simulink model "single_camera_xy_tracking"  (R2025b)
settings: Solver=FixedStepDiscrete  StartTime=0  StopTime=T_end  FixedStep=Ts  RelTol=1e-3
InitFcn:
  | init_single_camera_xy_tracking;
values from neighbouring files (symbols this model uses):
  controller_parameters = [      Ts; Z_hat; Kpx; Kpy; k_ff; gamma_adapt; sigma_adapt; adapt_max;      v_xy_max; a_xy_max; ekf_gate_threshold;      double(enable_proportional); double(enable_ekf_feedforward);      double(enable_adaptation); double(controller_enable);      ekf_reset_timeout_sec]    [init_single_camera_xy_tracking.m]
  cx = 1920    [init_single_camera_xy_tracking.m]
  cy = 1080    [init_single_camera_xy_tracking.m]
  fx = 800    [init_single_camera_xy_tracking.m]
  fy = 800    [init_single_camera_xy_tracking.m]
  joint_state_timeout_sec = 0.10    (= 0.1)    [init_single_camera_xy_tracking.m]
  P0 = diag([0.05^2, 0.05^2, 0.20^2, 0.20^2, 0.50^2, 0.50^2])    [init_single_camera_xy_tracking.m]
  pixel_noise_std = 0.8    [init_single_camera_xy_tracking.m]
  Q_ekf = diag([1e-6, 1e-6, 1e-4, 1e-4, 1e-2, 1e-2])    [init_single_camera_xy_tracking.m]
  R_ekf = diag([0.003^2, 0.003^2])    [init_single_camera_xy_tracking.m]
  random_seed_x = 1207    [init_single_camera_xy_tracking.m]
  random_seed_y = 9053    [init_single_camera_xy_tracking.m]
  target_timeout_sec = 0.20    (= 0.2)    [init_single_camera_xy_tracking.m]
  Ts = 0.01    [init_single_camera_xy_tracking.m]
  USE_ROS = true    [init_single_camera_xy_tracking.m]
  X0 = 0.45    [init_single_camera_xy_tracking.m]
  Y0 = -0.25    [init_single_camera_xy_tracking.m]
  Z0 = Z_hat    (= 0.75)    [init_single_camera_xy_tracking.m]
  Z_hat = 0.75    [init_single_camera_xy_tracking.m]
undefined symbols (not defined in the file or in its folder): data, data_SL_Info
libraries: ros2lib x4
Description:
  | Fixed-focus monocular XY target tracking. Outputs camera-frame [vx vy 0 0 0 0]; robot kinematics remain external.
settings Model: Creator=ASUS  LastModifiedBy=ASUS
settings DataIOCC: SignalLogging=off

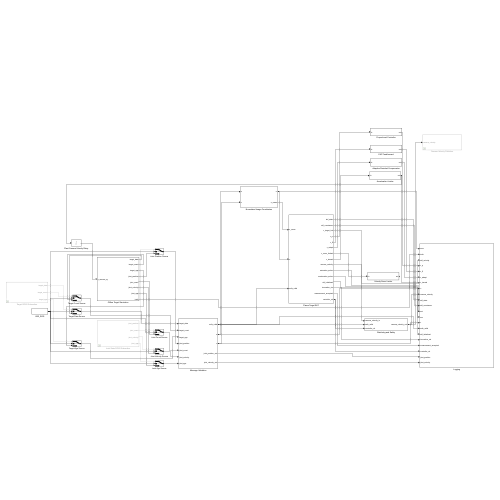
[thumbnail: Simulink's stored preview of the top-level diagram]
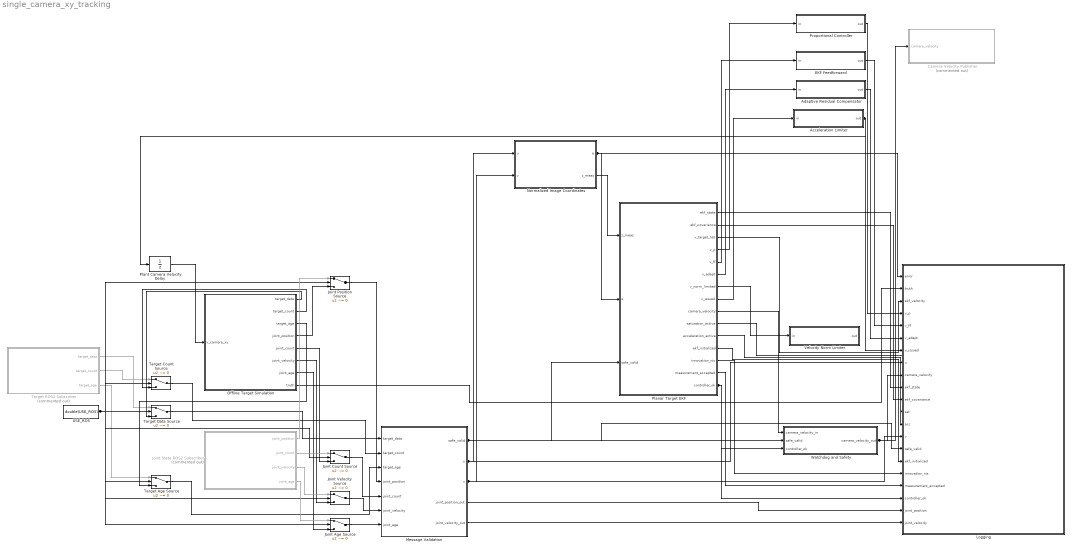
== system single_camera_xy_tracking ==
  Acceleration Limiter : Subsystem
  Adaptive Residual Compensator : Subsystem
  Camera Velocity Publisher : Subsystem  Commented=on
  EKF Feedforward : Subsystem
  Joint Age Source : Switch  Criteria=u2 ~= 0  Threshold=0.5  SaturateOnIntegerOverflow=off  InputSameDT=off
  Joint Count Source : Switch  Criteria=u2 ~= 0  Threshold=0.5  SaturateOnIntegerOverflow=off  InputSameDT=off
  Joint Position Source : Switch  Criteria=u2 ~= 0  Threshold=0.5  SaturateOnIntegerOverflow=off  InputSameDT=off
  Joint State ROS2 Subscriber : Subsystem  Commented=on
  Joint Velocity Source : Switch  Criteria=u2 ~= 0  Threshold=0.5  SaturateOnIntegerOverflow=off  InputSameDT=off
  Logging : Subsystem
  Message Validation : Subsystem
  Normalized Image Coordinates : Subsystem
  Offline Target Simulation : Subsystem
  Planar Target EKF : Subsystem
  Plant Camera Velocity Delay : UnitDelay  InitialCondition=[0;0]  SampleTime=Ts  HasFrameUpgradeWarning=on
  Proportional Controller : Subsystem
  Target Age Source : Switch  Criteria=u2 ~= 0  Threshold=0.5  SaturateOnIntegerOverflow=off  InputSameDT=off
  Target Count Source : Switch  Criteria=u2 ~= 0  Threshold=0.5  SaturateOnIntegerOverflow=off  InputSameDT=off
  Target Data Source : Switch  Criteria=u2 ~= 0  Threshold=0.5  SaturateOnIntegerOverflow=off  InputSameDT=off
  Target ROS2 Subscriber : Subsystem  Commented=on
  USE_ROS : Constant  Value=double(USE_ROS)
  Velocity Norm Limiter : Subsystem
  Watchdog and Safety : Subsystem
  wires:
  Target Age Source/1 -> Message Validation/3(target_age)
  Target Data Source/1 -> Message Validation/1(target_data)
  Target Count Source/1 -> Message Validation/2(target_count)
  Plant Camera Velocity Delay/1 -> Offline Target Simulation/1(v_camera_xy)
  Target ROS2 Subscriber/1(target_data) -> Target Data Source/1
  Planar Target EKF/3(v_target_hat) -> Logging/3(ekf_velocity)
  Message Validation/2(u) -> Logging/8(u), Normalized Image Coordinates/1(u)
  Target ROS2 Subscriber/2(target_count) -> Target Count Source/1
  Target ROS2 Subscriber/3(target_age) -> Target Age Source/1
  Planar Target EKF/15(controller_ok) -> Watchdog and Safety/3(controller_ok), Logging/19(controller_ok)
  Planar Target EKF/7(v_norm_limited) -> Velocity Norm Limiter/1(in)
  USE_ROS/1 -> Joint Age Source/2, Joint Velocity Source/2, Joint Position Source/2, Target Count Source/2, Joint Count Source/2, Target Data Source/2, Target Age Source/2
  Offline Target Simulation/1(target_data) -> Target Data Source/3
  Offline Target Simulation/2(target_count) -> Target Count Source/3
  Offline Target Simulation/3(target_age) -> Target Age Source/3
  Offline Target Simulation/4(joint_position) -> Joint Position Source/3
  Offline Target Simulation/5(joint_count) -> Joint Count Source/3
  Offline Target Simulation/6(joint_velocity) -> Joint Velocity Source/3
  Adaptive Residual Compensator/1(out) -> Logging/6(v_adapt)
  Offline Target Simulation/7(joint_age) -> Joint Age Source/3
  Offline Target Simulation/8(truth) -> Logging/2(truth)
  Joint Age Source/1 -> Message Validation/7(joint_age)
  Joint State ROS2 Subscriber/1(joint_position) -> Joint Position Source/1
  Joint Count Source/1 -> Message Validation/5(joint_count)
  Joint State ROS2 Subscriber/2(joint_count) -> Joint Count Source/1
  Joint Position Source/1 -> Message Validation/4(joint_position)
  Joint State ROS2 Subscriber/3(joint_velocity) -> Joint Velocity Source/1
  Joint State ROS2 Subscriber/4(joint_age) -> Joint Age Source/1
  Joint Velocity Source/1 -> Message Validation/6(joint_velocity)
  Planar Target EKF/4(v_p) -> Proportional Controller/1(in)
  Message Validation/1(safe_valid) -> Watchdog and Safety/2(safe_valid), Logging/15(safe_valid), Planar Target EKF/3(safe_valid)
  Message Validation/3(v) -> Logging/14(v), Normalized Image Coordinates/2(v)
  Planar Target EKF/5(v_ff) -> EKF Feedforward/1(in)
  Message Validation/4(joint_position_out) -> Logging/20(joint_position)
  Message Validation/5(joint_velocity_out) -> Logging/21(joint_velocity)
  Normalized Image Coordinates/1(e) -> Planar Target EKF/2(e), Logging/1(error)
  Normalized Image Coordinates/2(z_meas) -> Planar Target EKF/1(z_meas)
  Planar Target EKF/1(ekf_state) -> Logging/10(ekf_state)
  Planar Target EKF/2(ekf_covariance) -> Logging/11(ekf_covariance)
  Planar Target EKF/14(measurement_accepted) -> Logging/18(measurement_accepted)
  Planar Target EKF/6(v_adapt) -> Adaptive Residual Compensator/1(in)
  Planar Target EKF/8(v_issued) -> Acceleration Limiter/1(in)
  Planar Target EKF/10(saturation_active) -> Logging/12(sat)
  Planar Target EKF/11(acceleration_active) -> Logging/13(acc)
  Planar Target EKF/12(ekf_initialized) -> Logging/16(ekf_initialized)
  Planar Target EKF/13(innovation_nis) -> Logging/17(innovation_nis)
  Proportional Controller/1(out) -> Logging/4(v_p)
  EKF Feedforward/1(out) -> Logging/5(v_ff)
  Acceleration Limiter/1(out) -> Logging/7(v_issued), Plant Camera Velocity Delay/1
  Planar Target EKF/9(camera_velocity) -> Watchdog and Safety/1(camera_velocity_in)
  Watchdog and Safety/1(camera_velocity_out) -> Camera Velocity Publisher/1(camera_velocity), Logging/9(camera_velocity)

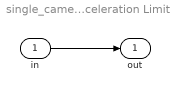
== system single_camera_xy_tracking/Acceleration Limiter ==
  in : Inport
  out : Outport
  wires:
  in/1 -> out/1

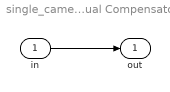
== system single_camera_xy_tracking/Adaptive Residual Compensator ==
  in : Inport
  out : Outport
  wires:
  in/1 -> out/1

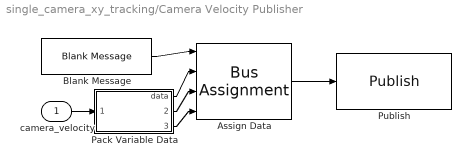
== system single_camera_xy_tracking/Camera Velocity Publisher ==
  camera_velocity : Inport
  Assign Data : BusAssignment  AssignedSignals=data,data_SL_Info.CurrentLength,data_SL_Info.ReceivedLength
  Blank Message : ros2lib/Blank Message  messageClass=Message  entityType=std_msgs/Float64MultiArray  messageType=std_msgs/Float64MultiArray  SampleTime=Ts
  Pack Variable Data : MATLAB Function  TreatAsAtomicUnit=on
  Publish : ros2lib/Publish  topicSource=Select from ROS network  topic=/simulink/camera_velocity  messageType=std_msgs/Float64MultiArray  QOSHistory=Keep last  QOSDepth=1  QOSReliability=Reliable  QOSDurability=Volatile  QOSDeadline=Inf  QOSLifespan=Inf  QOSLiveliness=Automatic  QOSLeaseDuration=Inf  QOSAvoidROSNamespaceConventions=off
  wires:
  Blank Message/1 -> Assign Data/1
  Assign Data/1 -> Publish/1
  camera_velocity/1 -> Pack Variable Data/1(camera_velocity)
  Pack Variable Data/1(data) -> Assign Data/2
  Pack Variable Data/2(current_length) -> Assign Data/3
  Pack Variable Data/3(received_length) -> Assign Data/4

== system single_camera_xy_tracking/EKF Feedforward ==
  in : Inport
  out : Outport
  wires:
  in/1 -> out/1

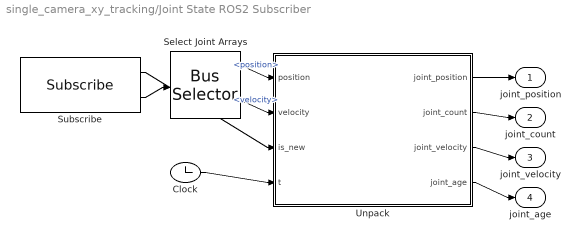
== system single_camera_xy_tracking/Joint State ROS2 Subscriber ==
  Clock : Clock
  Select Joint Arrays : BusSelector  OutputSignals=position,velocity
  Subscribe : ros2lib/Subscribe  topicSource=Select from ROS network  topic=/franka/joint_states  messageType=sensor_msgs/JointState  sampleTime=Ts  QOSHistory=Keep last  QOSDepth=1  QOSReliability=Best effort  QOSDurability=Volatile  QOSDeadline=Inf  QOSLifespan=Inf  QOSLiveliness=Automatic  QOSLeaseDuration=Inf  QOSAvoidROSNamespaceConventions=off
  Unpack : MATLAB Function  TreatAsAtomicUnit=on
  joint_position : Outport
  joint_count : Outport  Port=2
  joint_velocity : Outport  Port=3
  joint_age : Outport  Port=4
  wires:
  Unpack/1(joint_position) -> joint_position/1
  Unpack/2(joint_count) -> joint_count/1
  Unpack/3(joint_velocity) -> joint_velocity/1
  Unpack/4(joint_age) -> joint_age/1
  Select Joint Arrays/1 -> Unpack/1(position)  "<position>"
  Select Joint Arrays/2 -> Unpack/2(velocity)  "<velocity>"
  Clock/1 -> Unpack/4(t)
  Subscribe/2 -> Select Joint Arrays/1
  Subscribe/1 -> Unpack/3(is_new)

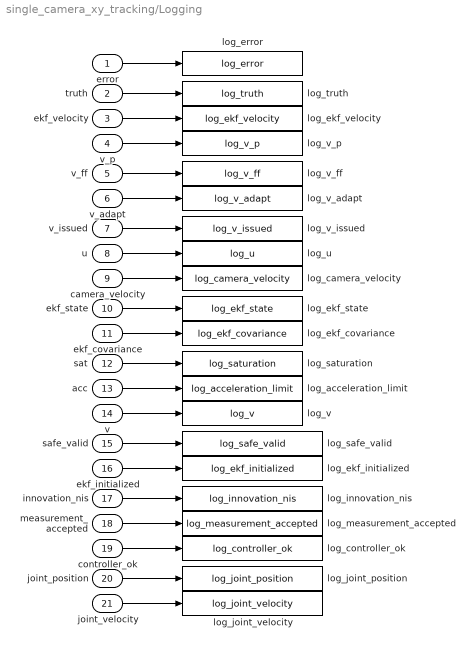
== system single_camera_xy_tracking/Logging ==
  error : Inport
  truth : Inport  Port=2
  ekf_velocity : Inport  Port=3
  v_p : Inport  Port=4
  v_ff : Inport  Port=5
  v_adapt : Inport  Port=6
  v_issued : Inport  Port=7
  u : Inport  Port=8
  camera_velocity : Inport  Port=9
  ekf_state : Inport  Port=10
  ekf_covariance : Inport  Port=11
  sat : Inport  Port=12
  acc : Inport  Port=13
  v : Inport  Port=14
  safe_valid : Inport  Port=15
  ekf_initialized : Inport  Port=16
  innovation_nis : Inport  Port=17
  measurement_accepted : Inport  Port=18
  controller_ok : Inport  Port=19
  joint_position : Inport  Port=20
  joint_velocity : Inport  Port=21
  log_acceleration_limit : ToWorkspace  VariableName=log_acceleration_limit  SaveFormat=Structure With Time  SampleTime=-1
  log_camera_velocity : ToWorkspace  VariableName=log_camera_velocity  SaveFormat=Structure With Time  SampleTime=-1
  log_controller_ok : ToWorkspace  VariableName=log_controller_ok  SaveFormat=Structure With Time  SampleTime=-1
  log_ekf_covariance : ToWorkspace  VariableName=log_ekf_covariance  SaveFormat=Structure With Time  SampleTime=-1
  log_ekf_initialized : ToWorkspace  VariableName=log_ekf_initialized  SaveFormat=Structure With Time  SampleTime=-1
  log_ekf_state : ToWorkspace  VariableName=log_ekf_state  SaveFormat=Structure With Time  SampleTime=-1
  log_ekf_velocity : ToWorkspace  VariableName=log_ekf_velocity  SaveFormat=Structure With Time  SampleTime=-1
  log_error : ToWorkspace  VariableName=log_error  SaveFormat=Structure With Time  SampleTime=-1
  log_innovation_nis : ToWorkspace  VariableName=log_innovation_nis  SaveFormat=Structure With Time  SampleTime=-1
  log_joint_position : ToWorkspace  VariableName=log_joint_position  SaveFormat=Structure With Time  SampleTime=-1
  log_joint_velocity : ToWorkspace  VariableName=log_joint_velocity  SaveFormat=Structure With Time  SampleTime=-1
  log_measurement_accepted : ToWorkspace  VariableName=log_measurement_accepted  SaveFormat=Structure With Time  SampleTime=-1
  log_safe_valid : ToWorkspace  VariableName=log_safe_valid  SaveFormat=Structure With Time  SampleTime=-1
  log_saturation : ToWorkspace  VariableName=log_saturation  SaveFormat=Structure With Time  SampleTime=-1
  log_truth : ToWorkspace  VariableName=log_truth  SaveFormat=Structure With Time  SampleTime=-1
  log_u : ToWorkspace  VariableName=log_u  SaveFormat=Structure With Time  SampleTime=-1
  log_v : ToWorkspace  VariableName=log_v  SaveFormat=Structure With Time  SampleTime=-1
  log_v_adapt : ToWorkspace  VariableName=log_v_adapt  SaveFormat=Structure With Time  SampleTime=-1
  log_v_ff : ToWorkspace  VariableName=log_v_ff  SaveFormat=Structure With Time  SampleTime=-1
  log_v_issued : ToWorkspace  VariableName=log_v_issued  SaveFormat=Structure With Time  SampleTime=-1
  log_v_p : ToWorkspace  VariableName=log_v_p  SaveFormat=Structure With Time  SampleTime=-1
  wires:
  error/1 -> log_error/1
  truth/1 -> log_truth/1
  ekf_velocity/1 -> log_ekf_velocity/1
  v_p/1 -> log_v_p/1
  v_ff/1 -> log_v_ff/1
  v_adapt/1 -> log_v_adapt/1
  v_issued/1 -> log_v_issued/1
  u/1 -> log_u/1
  camera_velocity/1 -> log_camera_velocity/1
  ekf_state/1 -> log_ekf_state/1
  ekf_covariance/1 -> log_ekf_covariance/1
  sat/1 -> log_saturation/1
  acc/1 -> log_acceleration_limit/1
  v/1 -> log_v/1
  safe_valid/1 -> log_safe_valid/1
  ekf_initialized/1 -> log_ekf_initialized/1
  innovation_nis/1 -> log_innovation_nis/1
  measurement_accepted/1 -> log_measurement_accepted/1
  controller_ok/1 -> log_controller_ok/1
  joint_position/1 -> log_joint_position/1
  joint_velocity/1 -> log_joint_velocity/1

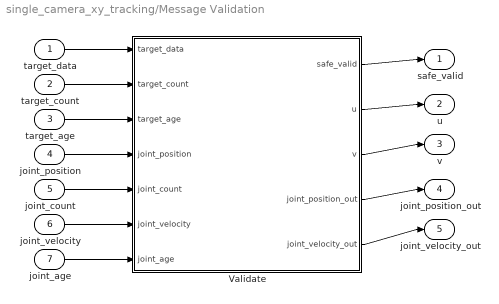
== system single_camera_xy_tracking/Message Validation ==
  target_data : Inport
  target_count : Inport  Port=2
  target_age : Inport  Port=3
  joint_position : Inport  Port=4
  joint_count : Inport  Port=5
  joint_velocity : Inport  Port=6
  joint_age : Inport  Port=7
  Validate : MATLAB Function  TreatAsAtomicUnit=on
  safe_valid : Outport
  u : Outport  Port=2
  v : Outport  Port=3
  joint_position_out : Outport  Port=4
  joint_velocity_out : Outport  Port=5
  wires:
  Validate/1(safe_valid) -> safe_valid/1
  Validate/2(u) -> u/1
  Validate/3(v) -> v/1
  Validate/4(joint_position_out) -> joint_position_out/1
  Validate/5(joint_velocity_out) -> joint_velocity_out/1
  target_data/1 -> Validate/1(target_data)
  target_count/1 -> Validate/2(target_count)
  target_age/1 -> Validate/3(target_age)
  joint_position/1 -> Validate/4(joint_position)
  joint_count/1 -> Validate/5(joint_count)
  joint_velocity/1 -> Validate/6(joint_velocity)
  joint_age/1 -> Validate/7(joint_age)

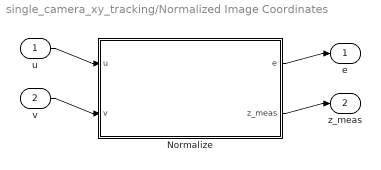
== system single_camera_xy_tracking/Normalized Image Coordinates ==
  u : Inport
  v : Inport  Port=2
  Normalize : MATLAB Function  TreatAsAtomicUnit=on
  e : Outport
  z_meas : Outport  Port=2
  wires:
  u/1 -> Normalize/1(u)
  v/1 -> Normalize/2(v)
  Normalize/1(e) -> e/1
  Normalize/2(z_meas) -> z_meas/1

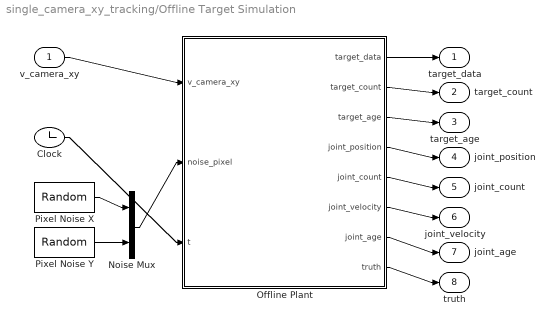
== system single_camera_xy_tracking/Offline Target Simulation ==
  v_camera_xy : Inport
  Clock : Clock
  Noise Mux : Mux  Inputs=2
  Offline Plant : MATLAB Function  TreatAsAtomicUnit=on
  Pixel Noise X : RandomNumber  Variance=pixel_noise_std^2  Seed=random_seed_x  SampleTime=Ts
  Pixel Noise Y : RandomNumber  Variance=pixel_noise_std^2  Seed=random_seed_y  SampleTime=Ts
  target_data : Outport
  target_count : Outport  Port=2
  target_age : Outport  Port=3
  joint_position : Outport  Port=4
  joint_count : Outport  Port=5
  joint_velocity : Outport  Port=6
  joint_age : Outport  Port=7
  truth : Outport  Port=8
  wires:
  Offline Plant/1(target_data) -> target_data/1
  Offline Plant/2(target_count) -> target_count/1
  Offline Plant/3(target_age) -> target_age/1
  Offline Plant/4(joint_position) -> joint_position/1
  Offline Plant/5(joint_count) -> joint_count/1
  Offline Plant/6(joint_velocity) -> joint_velocity/1
  Offline Plant/7(joint_age) -> joint_age/1
  Offline Plant/8(truth) -> truth/1
  v_camera_xy/1 -> Offline Plant/1(v_camera_xy)
  Pixel Noise X/1 -> Noise Mux/1
  Pixel Noise Y/1 -> Noise Mux/2
  Noise Mux/1 -> Offline Plant/2(noise_pixel)
  Clock/1 -> Offline Plant/3(t)

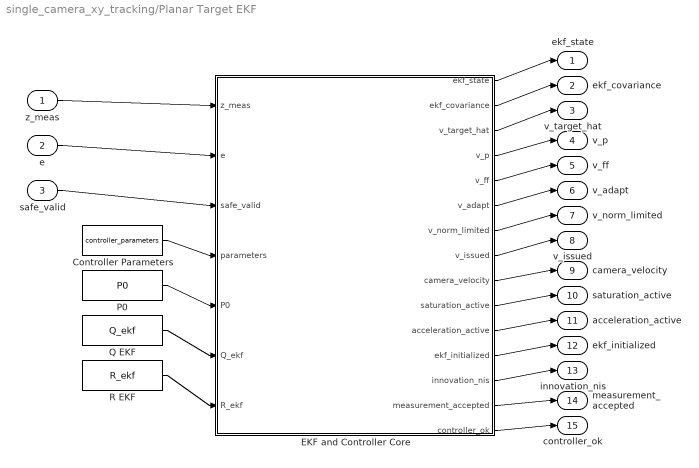
== system single_camera_xy_tracking/Planar Target EKF ==
  z_meas : Inport
  e : Inport  Port=2
  safe_valid : Inport  Port=3
  Controller Parameters : Constant  Value=controller_parameters
  EKF and Controller Core : MATLAB Function  TreatAsAtomicUnit=on
  P0 : Constant  Value=P0
  Q EKF : Constant  Value=Q_ekf
  R EKF : Constant  Value=R_ekf
  ekf_state : Outport
  ekf_covariance : Outport  Port=2
  v_target_hat : Outport  Port=3
  v_p : Outport  Port=4
  v_ff : Outport  Port=5
  v_adapt : Outport  Port=6
  v_norm_limited : Outport  Port=7
  v_issued : Outport  Port=8
  camera_velocity : Outport  Port=9
  saturation_active : Outport  Port=10
  acceleration_active : Outport  Port=11
  ekf_initialized : Outport  Port=12
  innovation_nis : Outport  Port=13
  measurement_accepted : Outport  Port=14
  controller_ok : Outport  Port=15
  wires:
  EKF and Controller Core/1(ekf_state) -> ekf_state/1
  EKF and Controller Core/2(ekf_covariance) -> ekf_covariance/1
  EKF and Controller Core/3(v_target_hat) -> v_target_hat/1
  EKF and Controller Core/4(v_p) -> v_p/1
  EKF and Controller Core/5(v_ff) -> v_ff/1
  EKF and Controller Core/6(v_adapt) -> v_adapt/1
  EKF and Controller Core/7(v_norm_limited) -> v_norm_limited/1
  EKF and Controller Core/8(v_issued) -> v_issued/1
  EKF and Controller Core/9(camera_velocity) -> camera_velocity/1
  EKF and Controller Core/10(saturation_active) -> saturation_active/1
  EKF and Controller Core/11(acceleration_active) -> acceleration_active/1
  EKF and Controller Core/12(ekf_initialized) -> ekf_initialized/1
  EKF and Controller Core/13(innovation_nis) -> innovation_nis/1
  EKF and Controller Core/14(measurement_accepted) -> measurement_accepted/1
  EKF and Controller Core/15(controller_ok) -> controller_ok/1
  z_meas/1 -> EKF and Controller Core/1(z_meas)
  e/1 -> EKF and Controller Core/2(e)
  safe_valid/1 -> EKF and Controller Core/3(safe_valid)
  Controller Parameters/1 -> EKF and Controller Core/4(parameters)
  P0/1 -> EKF and Controller Core/5(P0)
  Q EKF/1 -> EKF and Controller Core/6(Q_ekf)
  R EKF/1 -> EKF and Controller Core/7(R_ekf)

== system single_camera_xy_tracking/Proportional Controller ==
  in : Inport
  out : Outport
  wires:
  in/1 -> out/1

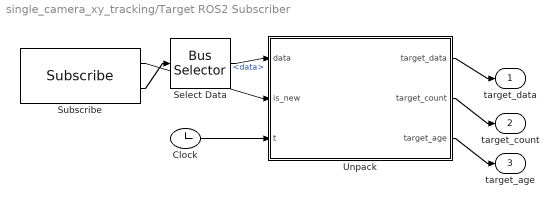
== system single_camera_xy_tracking/Target ROS2 Subscriber ==
  Clock : Clock
  Select Data : BusSelector  OutputSignals=data
  Subscribe : ros2lib/Subscribe  topicSource=Select from ROS network  topic=/apriltag_detector/target_position  messageType=std_msgs/Float64MultiArray  sampleTime=Ts  QOSHistory=Keep last  QOSDepth=1  QOSReliability=Best effort  QOSDurability=Volatile  QOSDeadline=Inf  QOSLifespan=Inf  QOSLiveliness=Automatic  QOSLeaseDuration=Inf  QOSAvoidROSNamespaceConventions=off
  Unpack : MATLAB Function  TreatAsAtomicUnit=on
  target_data : Outport
  target_count : Outport  Port=2
  target_age : Outport  Port=3
  wires:
  Unpack/1(target_data) -> target_data/1
  Unpack/2(target_count) -> target_count/1
  Unpack/3(target_age) -> target_age/1
  Select Data/1 -> Unpack/1(data)  "<data>"
  Clock/1 -> Unpack/3(t)
  Subscribe/2 -> Select Data/1
  Subscribe/1 -> Unpack/2(is_new)

== system single_camera_xy_tracking/Velocity Norm Limiter ==
  in : Inport
  out : Outport
  wires:
  in/1 -> out/1

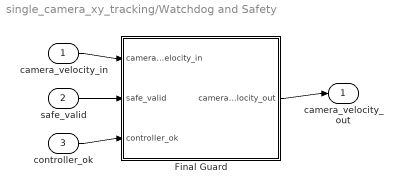
== system single_camera_xy_tracking/Watchdog and Safety ==
  camera_velocity_in : Inport
  safe_valid : Inport  Port=2
  controller_ok : Inport  Port=3
  Final Guard : MATLAB Function  TreatAsAtomicUnit=on
  camera_velocity_out : Outport
  wires:
  camera_velocity_in/1 -> Final Guard/1(camera_velocity_in)
  safe_valid/1 -> Final Guard/2(safe_valid)
  controller_ok/1 -> Final Guard/3(controller_ok)
  Final Guard/1(camera_velocity_out) -> camera_velocity_out/1

== matlab function single_camera_xy_tracking/Planar Target EKF/EKF and Controller Core ==
  data: z_meas input size=[2 1]; ekf_state output size=[6 1]; e input size=[2 1]; safe_valid input size=1; parameters input size=[16 1]; P0 input size=[6 6]; Q_ekf input size=[6 6]; R_ekf input size=[2 2]; ekf_covariance output size=[6 6]; v_target_hat output size=[2 1]; v_p output size=[2 1]; v_ff output size=[2 1]; v_adapt output size=[2 1]; v_norm_limited output size=[2 1]; v_issued output size=[2 1]; camera_velocity output size=[6 1]; saturation_active output size=1; acceleration_active output size=1; ekf_initialized output size=1; innovation_nis output size=1; measurement_accepted output size=1; controller_ok output size=1
function [ekf_state,ekf_covariance,v_target_hat,v_p,v_ff,v_adapt,v_norm_limited,v_issued,camera_velocity,saturation_active,acceleration_active,ekf_initialized,innovation_nis,measurement_accepted,controller_ok] = fcn(z_meas,e,safe_valid,parameters,P0,Q_ekf,R_ekf)
%#codegen
persistent x_hat P d_hat v_previous p_camera_hat invalid_time initialized
if isempty(initialized)
    x_hat=zeros(6,1); P=P0; d_hat=zeros(2,1); v_previous=zeros(2,1);
    p_camera_hat=zeros(2,1); invalid_time=0.0; initialized=false;
end
Ts=parameters(1); Z_hat=parameters(2); Kpx=parameters(3); Kpy=parameters(4);
k_ff=parameters(5); gamma=parameters(6); sigma=parameters(7); adapt_max=parameters(8);
v_max=parameters(9); a_max=parameters(10); gate=parameters(11);
enable_p=parameters(12)>0.5; enable_ff=parameters(13)>0.5; enable_adapt=parameters(14)>0.5;
controller_enable=parameters(15)>0.5; reset_timeout=parameters(16);
ekf_state=zeros(6,1); ekf_covariance=P0; v_target_hat=zeros(2,1);
v_p=zeros(2,1); v_ff=zeros(2,1); v_adapt=zeros(2,1);
v_norm_limited=zeros(2,1); v_issued=zeros(2,1); camera_velocity=zeros(6,1);
saturation_active=false; acceleration_active=false; ekf_initialized=initialized;
innovation_nis=0.0; measurement_accepted=false; controller_ok=false;
F=[1 0 Ts 0 0.5*Ts*Ts 0;0 1 0 Ts 0 0.5*Ts*Ts;0 0 1 0 Ts 0;0 0 0 1 0 Ts;0 0 0 0 1 0;0 0 0 0 0 1];
H=[1 0 0 0 0 0;0 1 0 0 0 0]; I6=eye(6);
p_camera_hat=p_camera_hat+Ts*v_previous;
parameter_ok=all(isfinite(parameters(:))) && Ts>0 && Z_hat>0 && v_max>0 && a_max>0 && reset_timeout>=Ts;
input_ok=safe_valid && controller_enable && parameter_ok && all(isfinite(z_meas(:))) && all(isfinite(e(:)));
if ~input_ok
    if initialized, x_hat=F*x_hat; P=F*P*F'+Q_ekf; P=0.5*(P+P'); end
    invalid_time=invalid_time+Ts; d_hat=zeros(2,1); v_previous=zeros(2,1);
    state_ok=all(isfinite(x_hat(:))) && all(isfinite(P(:))) && all(diag(P)>=0);
    if invalid_time>=reset_timeout || ~state_ok, x_hat=zeros(6,1); P=P0; initialized=false; end
    ekf_state=x_hat; ekf_covariance=P; v_target_hat=x_hat(3:4); ekf_initialized=initialized;
    return
end
invalid_time=0.0; z_ekf=z_meas+p_camera_hat;
if ~initialized
    x_hat=[z_ekf(1);z_ekf(2);0;0;0;0]; P=P0; initialized=true; measurement_accepted=true;
else
    x_pred=F*x_hat; P_pred=F*P*F'+Q_ekf; P_pred=0.5*(P_pred+P_pred');
    innovation=z_ekf-H*x_pred; S=H*P_pred*H'+R_ekf;
    if all(isfinite(S(:))) && rcond(S)>1e-12
        innovation_nis=innovation'*(S\innovation);
    else
        innovation_nis=inf;
    end
    x_hat=x_pred; P=P_pred;
    if isfinite(innovation_nis) && innovation_nis<=gate
        K=(P_pred*H')/S; x_hat=x_pred+K*innovation; A=I6-K*H;
        P=A*P_pred*A'+K*R_ekf*K'; P=0.5*(P+P'); measurement_accepted=true;
    end
end
ekf_ok=all(isfinite(x_hat(:))) && all(isfinite(P(:))) && all(diag(P)>=0) && norm(P-P','fro')<1e-6;
if ~ekf_ok
    x_hat=zeros(6,1); P=P0; d_hat=zeros(2,1); v_previous=zeros(2,1); p_camera_hat=zeros(2,1); initialized=false;
    return
end
ekf_state=x_hat; ekf_covariance=P; v_target_hat=x_hat(3:4); ekf_initialized=initialized;
if ~measurement_accepted
    d_hat=zeros(2,1); v_previous=zeros(2,1); return
end
if enable_p, v_p=Z_hat*[Kpx*e(1);Kpy*e(2)]; end
if enable_ff, v_ff=k_ff*v_target_hat; end
if enable_adapt
    leak=max(0.0,1.0-sigma*Ts); d_hat=leak*d_hat+gamma*Z_hat*e*Ts;
    d_hat(1)=min(max(d_hat(1),-adapt_max),adapt_max); d_hat(2)=min(max(d_hat(2),-adapt_max),adapt_max);
else
    d_hat=zeros(2,1);
end
v_adapt=d_hat; raw=v_p+v_ff+v_adapt; raw_norm=norm(raw);
saturation_active=raw_norm>v_max;
if saturation_active, v_norm_limited=raw*(v_max/raw_norm); else, v_norm_limited=raw; end
dv=v_norm_limited-v_previous; dv_norm=norm(dv); dv_max=a_max*Ts; acceleration_active=dv_norm>dv_max;
if acceleration_active, v_issued=v_previous+dv*(dv_max/dv_norm); else, v_issued=v_norm_limited; end
controller_ok=all(isfinite(v_p(:))) && all(isfinite(v_ff(:))) && all(isfinite(d_hat(:))) && all(isfinite(v_issued(:)));
if controller_ok
    v_previous=v_issued; camera_velocity=[v_issued;0;0;0;0];
else
    x_hat=zeros(6,1); P=P0; d_hat=zeros(2,1); v_previous=zeros(2,1); p_camera_hat=zeros(2,1); initialized=false;
    ekf_state=x_hat; ekf_covariance=P; v_target_hat=zeros(2,1); v_adapt=zeros(2,1); v_norm_limited=zeros(2,1); v_issued=zeros(2,1);
end
ekf_initialized=initialized;
end

== matlab function single_camera_xy_tracking/Watchdog and Safety/Final Guard ==
  data: camera_velocity_in input size=[6 1]; camera_velocity_out output size=[6 1]; safe_valid input size=1; controller_ok input size=1
function camera_velocity_out = fcn(camera_velocity_in,safe_valid,controller_ok)
%#codegen
camera_velocity_out=zeros(6,1);
if safe_valid && controller_ok && all(isfinite(camera_velocity_in(:)))
    camera_velocity_out=camera_velocity_in;
    camera_velocity_out(3:6)=0;
end
end

== matlab function single_camera_xy_tracking/Camera Velocity Publisher/Pack Variable Data ==
  data: camera_velocity input size=[6 1]; data output size=[128 1]; current_length output size=1; received_length output size=1
function [data,current_length,received_length] = fcn(camera_velocity)
%#codegen
data=zeros(128,1); data(1:6)=camera_velocity;
current_length=uint32(6); received_length=uint32(6);
end

== matlab function single_camera_xy_tracking/Target ROS2 Subscriber/Unpack ==
  data: data input; target_data output size=[3 1]; is_new input size=1; t input size=1; target_count output size=1; target_age output size=1
function [target_data,target_count,target_age] = fcn(data,is_new,t)
%#codegen
persistent last_data last_count last_time
if isempty(last_count), last_data=zeros(3,1); last_count=0.0; last_time=-1.0e6; end
if is_new
    n=numel(data); last_data=zeros(3,1);
    if n>=1, last_data(1)=data(1); end
    if n>=2, last_data(2)=data(2); end
    if n>=3, last_data(3)=data(3); end
    last_count=double(n); last_time=t;
end
target_data=last_data; target_count=last_count; target_age=max(0.0,t-last_time);
end

== matlab function single_camera_xy_tracking/Offline Target Simulation/Offline Plant ==
  data: v_camera_xy input size=[2 1]; target_data output size=[3 1]; noise_pixel input size=[2 1]; t input size=1; target_count output size=1; target_age output size=1; joint_position output size=[7 1]; joint_count output size=1; joint_velocity output size=[7 1]; joint_age output size=1; truth output size=[4 1]; Ts parameter size=1; fx parameter size=1; fy parameter size=1; cx parameter size=1; cy parameter size=1; Z0 parameter size=1; X0 parameter size=1; Y0 parameter size=1
function [target_data,target_count,target_age,joint_position,joint_count,joint_velocity,joint_age,truth] = fcn(v_camera_xy,noise_pixel,t, Ts, fx, fy, cx, cy, Z0, X0, Y0)
%#codegen
persistent X_state Y_state
if isempty(X_state), X_state=double(X0); end
if isempty(Y_state), Y_state=double(Y0); end
Vx_target=0.055*sin(0.55*t)+0.025;
Vy_target=0.045*cos(0.45*t)-0.015;
u=fx*X_state/Z0+cx+noise_pixel(1);
v=fy*Y_state/Z0+cy+noise_pixel(2);
target_data=zeros(3,1); target_data(1)=1.0; target_data(2)=u; target_data(3)=v; target_count=3.0; target_age=0.0;
joint_position=zeros(7,1); joint_count=7.0;
joint_velocity=zeros(7,1); joint_age=0.0;
truth=zeros(4,1); truth(1)=X_state; truth(2)=Y_state; truth(3)=Vx_target; truth(4)=Vy_target;
X_state=X_state+Ts*(Vx_target-v_camera_xy(1));
Y_state=Y_state+Ts*(Vy_target-v_camera_xy(2));
end

== matlab function single_camera_xy_tracking/Joint State ROS2 Subscriber/Unpack ==
  data: position input; joint_position output size=[7 1]; velocity input; is_new input size=1; t input size=1; joint_count output size=1; joint_velocity output size=[7 1]; joint_age output size=1
function [joint_position,joint_count,joint_velocity,joint_age] = fcn(position,velocity,is_new,t)
%#codegen
persistent last_q last_dq last_count last_time
if isempty(last_count), last_q=zeros(7,1); last_dq=zeros(7,1); last_count=0.0; last_time=-1.0e6; end
if is_new
    np=numel(position); nv=numel(velocity); last_q=zeros(7,1); last_dq=zeros(7,1);
    for k=1:min(np,7), last_q(k)=position(k); end
    for k=1:min(nv,7), last_dq(k)=velocity(k); end
    last_count=double(min(np,nv)); last_time=t;
end
joint_position=last_q; joint_count=last_count; joint_velocity=last_dq; joint_age=max(0.0,t-last_time);
end

== matlab function single_camera_xy_tracking/Message Validation/Validate ==
  data: target_data input size=[3 1]; safe_valid output size=1; target_count input size=1; target_age input size=1; joint_position input size=[7 1]; joint_count input size=1; joint_velocity input size=[7 1]; joint_age input size=1; u output size=1; v output size=1; joint_position_out output size=[7 1]; joint_velocity_out output size=[7 1]; target_timeout_sec parameter size=1; joint_state_timeout_sec parameter size=1
function [safe_valid,u,v,joint_position_out,joint_velocity_out] = fcn(target_data,target_count,target_age,joint_position,joint_count,joint_velocity,joint_age, target_timeout_sec, joint_state_timeout_sec)
%#codegen
u=0.0; v=0.0; joint_position_out=zeros(7,1); joint_velocity_out=zeros(7,1);
target_ok=target_count>=3 && target_data(1)>0.5 && isfinite(target_data(2)) && isfinite(target_data(3)) && isfinite(target_age) && target_age<=target_timeout_sec;
joint_ok=joint_count>=7 && all(isfinite(joint_position(:))) && all(isfinite(joint_velocity(:))) && isfinite(joint_age) && joint_age<=joint_state_timeout_sec;
if target_ok, u=target_data(2); v=target_data(3); end
if joint_ok, joint_position_out=joint_position; joint_velocity_out=joint_velocity; end
safe_valid=target_ok && joint_ok;
end

== matlab function single_camera_xy_tracking/Normalized Image Coordinates/Normalize ==
  data: u input size=1; e output size=[2 1]; v input size=1; z_meas output size=[2 1]; fx parameter size=1; fy parameter size=1; cx parameter size=1; cy parameter size=1; Z_hat parameter size=1
function [e,z_meas] = fcn(u,v, fx, fy, cx, cy, Z_hat)
%#codegen
ex=(u-cx)/fx; ey=(v-cy)/fy;
e=[ex;ey]; z_meas=Z_hat*e;
end
